simulink model "Controls_Model"  (R2024b)
settings: Solver=VariableStepAuto  StartTime=0.0  StopTime=10.0  RelTol=1e-3
undefined symbols (not defined in the file or in its folder): p
libraries: shared6dof x1
settings Model: Creator=gtanu  LastModifiedBy=gtanu

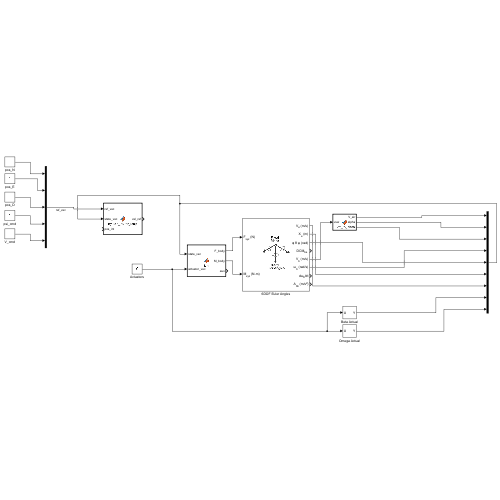
[thumbnail: Simulink's stored preview of the top-level diagram]
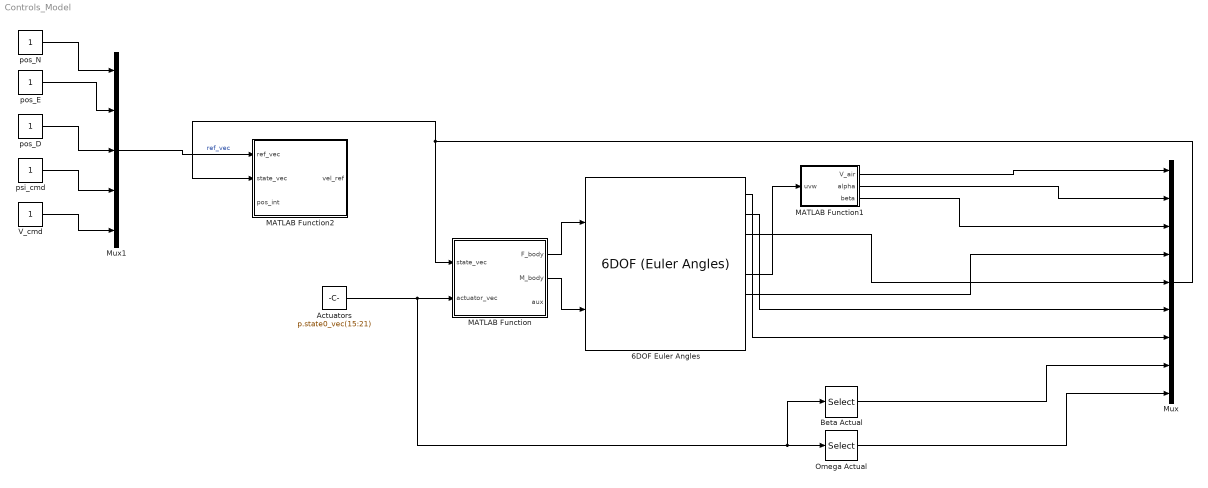
== system Controls_Model ==
  6DOF Euler Angles : shared6dof/6DOF (Euler Angles)  units=Metric (MKS)  mtype=Fixed  rep=Euler Angles  xme_0=[0 0 0]  Vm_0=[0 0 0]  eul_0=[0 0 0]  pm_0=[0 0 0]  mass_0=1.0  mass_e=0.5  mass_f=2.0  inertia=eye(3)  inertia_e=eye(3)  inertia_f=2*eye(3)  k_quat=1.0  vre_flag=on  abi_flag=off  aMode=0  xme_statename=''  Vm_statename=''  eul_statename=''  quat_statename=''  pm_statename=''  mass_statename=''
  Actuators : Constant  Value=p.state0_vec(15:21)
  Beta Actual : Selector  InputPortWidth=7  IndexOptions=Index vector (dialog)  Indices=[6 7]  OutputSizes=1
  MATLAB Function : MATLAB Function  TreatAsAtomicUnit=on
  MATLAB Function1 : MATLAB Function  TreatAsAtomicUnit=on
  MATLAB Function2 : MATLAB Function  TreatAsAtomicUnit=on
  Mux : Mux  Inputs=9
  Mux1 : Mux  Inputs=5
  Omega Actual : Selector  InputPortWidth=7  IndexOptions=Index vector (dialog)  Indices=[1 5]  OutputSizes=1
  V_cmd : Constant
  pos_D : Constant
  pos_E : Constant
  pos_N : Constant
  psi_cmd : Constant
  wires:
  Actuators/1 -> Beta Actual/1, Omega Actual/1, MATLAB Function/2(actuator_vec)
  Mux/1 -> MATLAB Function/1(state_vec), MATLAB Function2/2(state_vec)
  Beta Actual/1 -> Mux/8
  Omega Actual/1 -> Mux/9
  6DOF Euler Angles/5 -> MATLAB Function1/1(uvw)
  MATLAB Function1/1(V_air) -> Mux/1
  MATLAB Function1/2(alpha) -> Mux/2
  MATLAB Function1/3(beta) -> Mux/3
  6DOF Euler Angles/6 -> Mux/4
  6DOF Euler Angles/3 -> Mux/5
  6DOF Euler Angles/2 -> Mux/6
  6DOF Euler Angles/1 -> Mux/7
  MATLAB Function/1(F_body) -> 6DOF Euler Angles/1
  MATLAB Function/2(M_body) -> 6DOF Euler Angles/2
  pos_N/1 -> Mux1/1
  pos_E/1 -> Mux1/2
  pos_D/1 -> Mux1/3
  psi_cmd/1 -> Mux1/4
  V_cmd/1 -> Mux1/5
  Mux1/1 -> MATLAB Function2/1(ref_vec)  "ref_vec"

== matlab function Controls_Model/MATLAB Function1 ==
  data: uvw input; V_air output; alpha output; beta output
function [V_air, alpha, beta] = uvw_to_aero(uvw)
%#codegen
u = uvw(1); v = uvw(2); w = uvw(3);
V_air = sqrt(u^2 + v^2 + w^2);
V_air = max(V_air, 0.1);
alpha = atan2(w, u);
beta  = asin(v / V_air);

== matlab function Controls_Model/MATLAB Function ==
  data: state_vec input; F_body output; actuator_vec input; M_body output; aux output
function [F_body, M_body,aux] = fcn(state_vec, actuator_vec)
%#codegen
% state_vec:    21×1  (see dyulon_init section 15 for index definitions)
% actuator_vec:  7×1  [Omega_FL, Omega_FR, Omega_RL, Omega_RR, 
%                       beta_FL, beta_FR, delta_ail]

% --- Unpack only what forces_moments needs ---
state.V_air     = state_vec(1);
state.alpha     = state_vec(2);
state.beta_side = state_vec(3);
state.p_rate    = state_vec(4);
state.q_rate    = state_vec(5);
state.r_rate    = state_vec(6);
% [7:15] attitude and position — not needed by forces_moments
% [16:21] actuator feedback — not needed by forces_moments

% --- Unpack actuators ---
actuators.Omega(1)  = actuator_vec(1);   % Omega_FL
actuators.Omega(2)  = actuator_vec(2);   % Omega_FR
actuators.Omega(3)  = actuator_vec(3);   % Omega_RL
actuators.Omega(4)  = actuator_vec(4);   % Omega_RR
actuators.beta(1)   = actuator_vec(5);   % beta_FL
actuators.beta(2)   = actuator_vec(6);   % beta_FR
actuators.delta_ail = actuator_vec(7);

% --- Call physics ---
%DYULON_FORCES_MOMENTS  Compute total forces and moments on the Dyulon airframe.
%  Rev 4 - rear motors now independently tilt (pusher convention, beta=0=down)
%
%  REV 4 CHANGES:
%    - p.has_tilt is now [1,1,1,1] - all four motors tilt
%    - Rear motors use a DIFFERENT local beta convention than front:
%        Front: beta=0 -> up,   -90 -> forward (tractor)
%        Rear:  beta=0 -> down, -90 -> forward (pusher)
%      But the THRUST VECTOR FORMULA IS IDENTICAL for both:
%        T_vec_i = T_i * [-sin(beta_i); 0; -cos(beta_i)]
%      This works because the rear motor's beta is already measured from
%      its own local zero (straight-down), so the formula naturally
%      produces the correct physical force direction in the body frame.
%      No sign flip, no conditional logic needed.
%    - actuators.beta is now a 4-element vector [FL, FR, RL, RR]
%      (was previously 2-element front-only in Rev 3)
%    - p.beta_rear_fixed is no longer used; removed.
%
%  INPUTS:
%    state.V_air, .alpha, .beta_side, .p_rate, .q_rate, .r_rate
%    actuators.Omega(4), .beta(4), .delta_ail
%    p  - parameter struct from dyulon_init.m Rev 4
%
%  OUTPUTS:
%    F_body  [3x1]  total force  in body frame  [Fx; Fy; Fz]  N
%    M_body  [3x1]  total moment in body frame  [Mx; My; Mz]  N·m
%    aux     struct of intermediate quantities for logging/debug

V      = state.V_air;
alpha  = state.alpha;
beta_s = state.beta_side;
p_rate = state.p_rate;
q_rate = state.q_rate;
r_rate = state.r_rate;

q_bar = 0.5 * p.rho * max(V, 0.1)^2;

%% =========================================================================
%  A. PROPELLER FORCES AND MOMENTS
%% =========================================================================
F_prop = zeros(3,1);
M_prop = zeros(3,1);
M_gyro = zeros(3,1);

V_clamped = min(V, p.prop_V_bp(end));

scale_front = interp1(p.prop_V_bp, p.KpT_front_scale, V_clamped, 'linear');
KpT_front   = p.KpT_front_0 * scale_front;
KpM_front   = p.KpM_front_0 * scale_front;

scale_rear  = interp1(p.prop_V_bp, p.KpT_rear_scale,  V_clamped, 'linear');
KpT_rear    = p.KpT_rear_0  * scale_rear;
KpM_rear    = p.KpM_rear_0  * scale_rear;

% Approximate per-rotor inertia (spinner + blades, kg·m²)
I_rotor = 1.5e-4;
omega_body = [p_rate; q_rate; r_rate];

for i = 1:4
    Omega_i = actuators.Omega(i);

    if p.motor_type(i) == 1
        KpT_i = KpT_front;  KpM_i = KpM_front;
    else
        KpT_i = KpT_rear;   KpM_i = KpM_rear;
    end

    T_i = KpT_i * Omega_i^2;
    Q_i = KpM_i * Omega_i^2;

    % REV4: all motors now have independent tilt angle from actuators.beta(i)
    % Front motors: beta measured from straight-up    (0=up,   -90=fwd)
    % Rear  motors: beta measured from straight-down  (0=down, -90=fwd)
    % The formula below is IDENTICAL for both - convention baked into beta.
    beta_i = actuators.beta(i);

    % Thrust vector in body frame (x-forward, y-right, z-down):
    %   beta=0 front -> [-sin0; 0; -cos0]   = [0; 0; -1]*T -> up       (correct)
    %   beta=-90 any -> [-sin-90; 0; -cos-90] = [1; 0; 0]*T -> forward  (correct)
    %   beta=0 rear  -> [-sin0; 0; -cos0]   = [0; 0; -1]*T -> up?
    %   Wait: rear beta=0 is straight DOWN by convention, but formula gives
    %   [0;0;-T] which is UP. This is correct because T_i is the thrust
    %   reaction on the vehicle - the prop blows air down, vehicle goes UP.
    %   At beta_rear=-90: [1;0;0]*T = forward.  Correct.
    T_vec = T_i * [-sin(beta_i); 0; -cos(beta_i)];

    % Reaction torque along thrust axis (opposes spin direction)
    Q_vec = -p.spin_dir(i) * Q_i * [-sin(beta_i); 0; -cos(beta_i)];

    r_i = p.r_motor(i,:)';

    F_prop = F_prop + T_vec;
    M_prop = M_prop + cross(r_i, T_vec) + Q_vec;

    % Gyroscopic coupling: H = I_rotor * Omega * spin_axis
    spin_axis = [-sin(beta_i); 0; -cos(beta_i)];
    H_rotor   = p.spin_dir(i) * I_rotor * Omega_i * spin_axis;
    M_gyro    = M_gyro + cross(omega_body, H_rotor);
end

%% =========================================================================
%  B. WING AERODYNAMICS
%% =========================================================================
if V > 2.0
    alpha_deg     = rad2deg(alpha);
    alpha_clamped = max(p.aero_alpha_deg(1), min(p.aero_alpha_deg(end), alpha_deg));

    CL = interp1(p.aero_alpha_deg, p.aero_CL, alpha_clamped, 'linear');
    CD = interp1(p.aero_alpha_deg, p.aero_CD, alpha_clamped, 'linear');
    Cm = interp1(p.aero_alpha_deg, p.aero_Cm, alpha_clamped, 'linear');

    Lift = q_bar * p.S * CL;
    Drag = q_bar * p.S * CD;

    % Resolve lift/drag from wind frame to body frame
    Fx_aero =  Lift * sin(alpha) - Drag * cos(alpha);
    Fz_aero = -Lift * cos(alpha) - Drag * sin(alpha);
    % Side force - approximate, no vertical fin (Cy ≈ -0.15 per rad sideslip)
    Fy_aero =  q_bar * p.S * (-0.15) * beta_s;

    F_aero = [Fx_aero; Fy_aero; Fz_aero];

    % Pitch moment: aero Cm + pitch-rate damping
    Cm_total = Cm + p.Cm_q * (q_rate * p.cbar / (2 * max(V, 0.1)));
    My_aero  = q_bar * p.S * p.cbar * Cm_total;

    % Roll moment: dihedral + roll-rate damping + aileron
    Cl_total = p.Cl_b  * beta_s ...
             + p.Cl_p  * (p_rate * p.b / (2 * max(V, 0.1))) ...
             + p.Cl_da * actuators.delta_ail;
    Mx_aero  = q_bar * p.S * p.b * Cl_total;

    % Yaw moment: weathercock (weak, no fin) + yaw-rate damping
    Cn_total = p.Cn_b * beta_s + p.Cn_r * (r_rate * p.b / (2 * max(V, 0.1)));
    Mz_aero  = q_bar * p.S * p.b * Cn_total;

    M_aero = [Mx_aero; My_aero; Mz_aero];
else
    % Below 2 m/s aerodynamics are negligible and numerics get noisy
    F_aero = zeros(3,1);  M_aero = zeros(3,1);
    CL = 0; CD = 0; Cm = 0; Lift = 0; Drag = 0;
end

%% =========================================================================
%  C. TOTAL FORCES AND MOMENTS
%  NOTE: Gravity handled by Aerospace Blockset 6DOF (Euler Angles) block
%  internally in NED frame. Do NOT add gravity here.
%% =========================================================================
F_body = F_prop + F_aero;
M_body = M_prop + M_aero + M_gyro;

%% =========================================================================
%  D. AUX STRUCT (for Simulink logging and To Workspace blocks)
%% =========================================================================
aux.F_prop    = F_prop;
aux.F_aero    = F_aero;
aux.M_prop    = M_prop;
aux.M_aero    = M_aero;
aux.M_gyro    = M_gyro;
aux.KpT_front = KpT_front;
aux.KpT_rear  = KpT_rear;
aux.q_bar     = q_bar;
aux.CL        = CL;
aux.CD        = CD;
aux.Lift      = Lift;
aux.Drag      = Drag;

== matlab function Controls_Model/MATLAB Function2 ==
  data: ref_vec input; vel_ref output; state_vec input; pos_int input
function vel_ref = dyulon_outer_loop(ref_vec, state_vec, pos_int)
%DYULON_OUTER_LOOP  Position controller (outer loop).
%  Converts position error into a velocity reference command.
%
%  INPUTS:
%    ref_vec   [5x1]  [pos_N; pos_E; pos_D; psi_cmd; V_cmd]
%    state_vec [23x1] full state vector (see dyulon_init section 19)
%    pos_int   [3x1]  integrated position error from external Discrete
%                     Integrator block (Simulink), NOT computed here.
%                     Anti-windup saturation applied at the Simulink block
%                     level using p.gains.windup_limit_outer.
%
%  OUTPUTS:
%    vel_ref   [3x1]  [vN_ref; vE_ref; vD_ref]  m/s  NED frame
%
%  DESIGN NOTES:
%    - Pure PI on position. Ki starts at 0 (see dyulon_init) to avoid
%      windup during transition; raise only if steady-state position error
%      is unacceptable in simulation.
%    - Velocity commands are saturated before output. Saturation limits
%      are defined here as local constants because they are purely a
%      flight-envelope safety bound (not a tuning parameter), but they
%      reference p.V_stall_actual implicitly (max horizontal speed kept
%      well below stall).
%    - Integral state (pos_int) lives outside this function as a Simulink
%      Discrete Integrator block. This function only reads it.
%
%  STATE VECTOR INDEX REFERENCE (from dyulon_init section 19):
%    [10] pos_N  [11] pos_E  [12] pos_D
%    [13] vel_N  [14] vel_E  [15] vel_D
%#codegen

% --- Read gains from base workspace p struct ---
% (p is loaded by dyulon_init.m before simulation starts)
coder.extrinsic('evalin');
p = evalin('base', 'p');

% --- Unpack reference ---
pos_N_ref = ref_vec(1);
pos_E_ref = ref_vec(2);
pos_D_ref = ref_vec(3);
% ref_vec(4) = psi_cmd  - used by inner loop directly, not here
% ref_vec(5) = V_cmd    - used by inner loop directly, not here

% --- Unpack state (position) ---
pos_N = state_vec(10);
pos_E = state_vec(11);
pos_D = state_vec(12);

% --- Position error (NED) ---
err_N = pos_N_ref - pos_N;
err_E = pos_E_ref - pos_E;
err_D = pos_D_ref - pos_D;

% --- PI control ---
% Integral term (pos_int) fed in from external Simulink Discrete Integrator
vN_ref = p.gains.outer.Kp_xy * err_N + p.gains.outer.Ki_xy * pos_int(1);
vE_ref = p.gains.outer.Kp_xy * err_E + p.gains.outer.Ki_xy * pos_int(2);
vD_ref = p.gains.outer.Kp_z  * err_D + p.gains.outer.Ki_z  * pos_int(3);

% --- Output saturation ---
% Horizontal: keep well below stall (stall ~20 m/s, cap at 8 m/s for safety)
% Vertical: rate of climb target is 2 m/s from spec; cap descent at 3 m/s
vel_max_xy =  8.0;   % m/s
vel_max_dn =  3.0;   % m/s (positive = descend in NED)
vel_max_up = -2.0;   % m/s (negative = climb in NED)

vN_ref = max(min(vN_ref,  vel_max_xy), -vel_max_xy);
vE_ref = max(min(vE_ref,  vel_max_xy), -vel_max_xy);
vD_ref = max(min(vD_ref,  vel_max_dn),  vel_max_up);

vel_ref = [vN_ref; vE_ref; vD_ref];
